simulink model "DAC_Simscape"  (R2015b)
settings: Solver=VariableStepAuto  StartTime=0.0  StopTime=512  RelTol=1e-3
libraries: fl_lib x20, nesl_utility x10, elec_lib x8
settings Model: Creator=mihai.ciobanu  LastModifiedBy=mihai.ciobanu

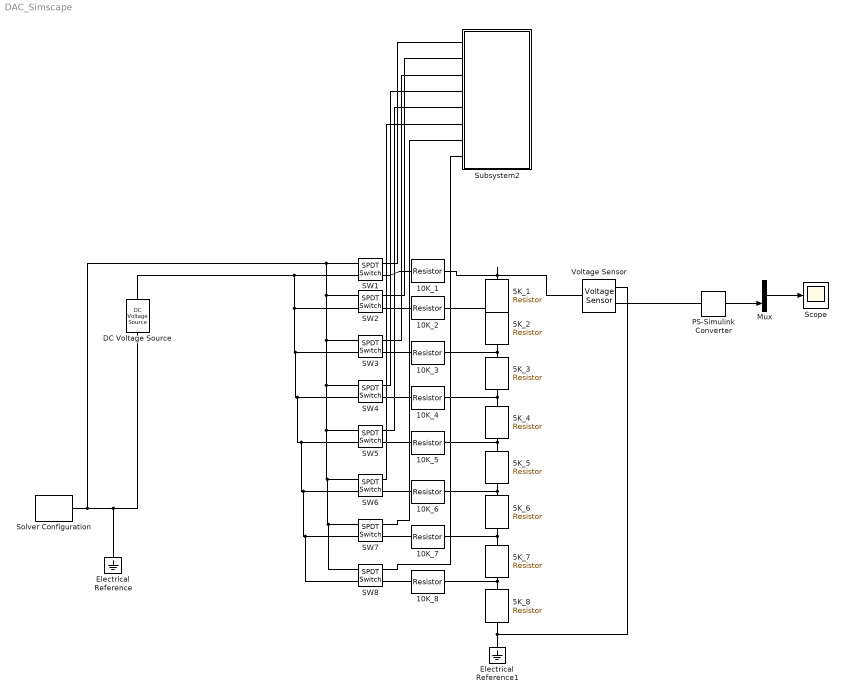
== system DAC_Simscape ==
  10K_{1..8} (8 alike) : fl_lib/Electrical/Electrical Elements/Resistor  R=10 kOhm  i_specify=off  i_priority=None  i=0 A  v_specify=off  v_priority=None  v=0 V
  5K_{1..8} (8 alike) : fl_lib/Electrical/Electrical Elements/Resistor  R=5 kOhm  i_specify=off  i_priority=None  i=0 A  v_specify=off  v_priority=None  v=0 V
  DC Voltage Source : fl_lib/Electrical/Electrical Sources/DC Voltage Source  v0=5 V
  Electrical Reference : fl_lib/Electrical/Electrical Elements/Electrical Reference
  Electrical Reference1 : fl_lib/Electrical/Electrical Elements/Electrical Reference
  Mux : Mux  Inputs=2
  PS-Simulink Converter : nesl_utility/PS-Simulink Converter  PhysicalDomain=network_engine_domain  SubClassName=ps_output  LeftPortType=input  RightPortType=output  PseudoPeriodic=off  Frequencies=[]  Unit=1  AffineConversion=off
  SW{1..8} (8 alike) : elec_lib/Passive Devices/Switches/SPDT Switch  R_closed=0.01 Ohm  G_open=1e-6 S  Threshold=0 V  Width=0 V  model_dynamics=0  t_on=0.001 s  t_off=0.001 s  initial_vT=0 V
  Scope : Scope
  Solver Configuration : nesl_utility/Solver Configuration  PhysicalDomain=network_engine_domain  SubClassName=solver  LeftPortType=input  RightPortType=generic  Accelerate=off  Tones=[]  Harmonics=[]  SimulateNoise=off  Profile=off  UseLocalSampling=off  EnableSwitchedLinearOptims=on  FrequencyDomain=off  UseCCode=off  RelTol=0.001  AbsTol=1e-06  MinStep=1e-09  ToWorkspace=off  RevertToSquareIcSolve=off  NumHomotopyIterations=100  PhasorMode=off  PhasorModeNumHarmonics=1  DoDC=off  ResidualTolerance=1e-09  UseLocalSolver=off  LocalSolverChoice=NE_BACKWARD_EULER_ADVANCER  LocalSolverSampleTime=0.001  DoFixedCost=off  MaxNonlinIter=3  MaxModeIter=2  LinearAlgebra=Sparse  DelaysMemoryBudget=1024  AutomaticFiltering=on  FilteringTimeConstant=0.001
  Subsystem2 : Subsystem
  Voltage Sensor : fl_lib/Electrical/Electrical Sensors/Voltage Sensor
  wires:
  PS-Simulink Converter/1 -> Mux/2
  Mux/1 -> Scope/1
  connections:
  SW1/RConn1 -- DC Voltage Source/RConn1 -- Electrical Reference/LConn1 -- Solver Configuration/RConn1 -- SW8/RConn1 -- SW7/RConn1 -- SW6/RConn1 -- SW5/RConn1 -- SW4/RConn1 -- SW3/RConn1 -- SW2/RConn1
  5K_1/RConn1 -- 5K_2/LConn1 -- 10K_2/RConn1
  5K_6/LConn1 -- 10K_6/RConn1 -- 5K_5/RConn1
  5K_3/LConn1 -- 10K_3/RConn1 -- 5K_2/RConn1
  5K_3/RConn1 -- 5K_4/LConn1 -- 10K_4/RConn1
  5K_4/RConn1 -- 10K_5/RConn1 -- 5K_5/LConn1
  5K_6/RConn1 -- 10K_7/RConn1 -- 5K_7/LConn1
  5K_7/RConn1 -- 10K_8/RConn1 -- 5K_8/LConn1
  Electrical Reference1/LConn1 -- Voltage Sensor/RConn2 -- 5K_8/RConn1
  10K_1/LConn1 -- SW1/LConn2
  SW2/LConn2 -- 10K_2/LConn1
  SW3/LConn2 -- 10K_3/LConn1
  10K_4/LConn1 -- SW4/LConn2
  SW5/LConn2 -- 10K_5/LConn1
  10K_6/LConn1 -- SW6/LConn2
  10K_7/LConn1 -- SW7/LConn2
  10K_8/LConn1 -- SW8/LConn2
  SW1/RConn2 -- DC Voltage Source/LConn1 -- SW8/RConn2 -- SW7/RConn2 -- SW6/RConn2 -- SW5/RConn2 -- SW4/RConn2 -- SW3/RConn2 -- SW2/RConn2
  5K_1/LConn1 -- Voltage Sensor/LConn1 -- 10K_1/RConn1
  Voltage Sensor/RConn1 -- PS-Simulink Converter/LConn1
  Subsystem2/RConn1 -- SW1/LConn1
  Subsystem2/RConn2 -- SW2/LConn1
  Subsystem2/RConn3 -- SW3/LConn1
  Subsystem2/RConn4 -- SW4/LConn1
  Subsystem2/RConn5 -- SW5/LConn1
  Subsystem2/RConn6 -- SW6/LConn1
  Subsystem2/RConn7 -- SW7/LConn1
  Subsystem2/RConn8 -- SW8/LConn1

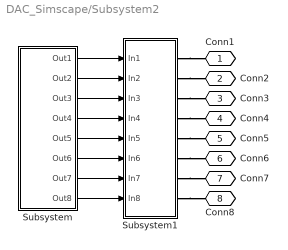
== system DAC_Simscape/Subsystem2 ==
  Subsystem : Subsystem
  Subsystem1 : Subsystem
  Conn1 : PMIOPort  Port=1  Side=Right
  Conn2 : PMIOPort  Port=2  Side=Right
  Conn3 : PMIOPort  Port=3  Side=Right
  Conn4 : PMIOPort  Port=4  Side=Right
  Conn5 : PMIOPort  Port=5  Side=Right
  Conn6 : PMIOPort  Port=6  Side=Right
  Conn7 : PMIOPort  Port=7  Side=Right
  Conn8 : PMIOPort  Port=8  Side=Right
  wires:
  Subsystem/5(Out5) -> Subsystem1/5(In5)
  Subsystem/4(Out4) -> Subsystem1/4(In4)
  Subsystem/1(Out1) -> Subsystem1/1(In1)
  Subsystem/7(Out7) -> Subsystem1/7(In7)
  Subsystem/6(Out6) -> Subsystem1/6(In6)
  Subsystem/8(Out8) -> Subsystem1/8(In8)
  Subsystem/2(Out2) -> Subsystem1/2(In2)
  Subsystem/3(Out3) -> Subsystem1/3(In3)
  connections:
  Subsystem1/RConn1 -- Conn1/RConn1
  Subsystem1/RConn3 -- Conn3/RConn1
  Subsystem1/RConn2 -- Conn2/RConn1
  Subsystem1/RConn4 -- Conn4/RConn1
  Subsystem1/RConn7 -- Conn7/RConn1
  Subsystem1/RConn8 -- Conn8/RConn1
  Subsystem1/RConn5 -- Conn5/RConn1
  Subsystem1/RConn6 -- Conn6/RConn1

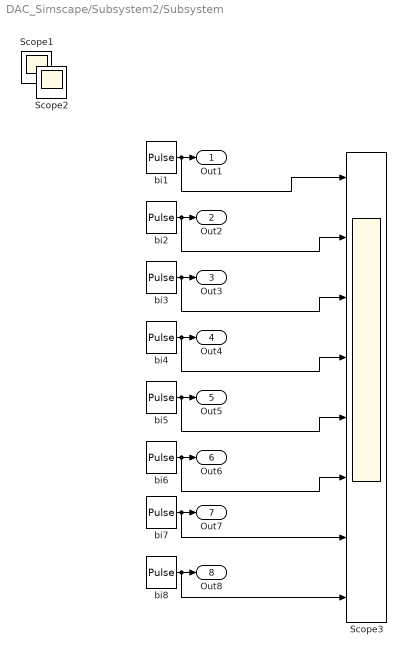
== system DAC_Simscape/Subsystem2/Subsystem ==
  Scope1 : Scope
  Scope2 : Scope
  Scope3 : Scope  NumInputPorts=8
  bi1 : DiscretePulseGenerator  PulseType=Time based  Period=256  PulseWidth=50
  bi2 : DiscretePulseGenerator  PulseType=Time based  Period=128  PulseWidth=50
  bi3 : DiscretePulseGenerator  PulseType=Time based  Period=64  PulseWidth=50
  bi4 : DiscretePulseGenerator  PulseType=Time based  Period=32  PulseWidth=50
  bi5 : DiscretePulseGenerator  PulseType=Time based  Period=16  PulseWidth=50
  bi6 : DiscretePulseGenerator  PulseType=Time based  Period=8  PulseWidth=50
  bi7 : DiscretePulseGenerator  PulseType=Time based  Period=4  PulseWidth=50
  bi8 : DiscretePulseGenerator  PulseType=Time based  PulseWidth=50
  Out1 : Outport
  Out2 : Outport  Port=2
  Out3 : Outport  Port=3
  Out4 : Outport  Port=4
  Out5 : Outport  Port=5
  Out6 : Outport  Port=6
  Out7 : Outport  Port=7
  Out8 : Outport  Port=8
  wires:
  bi1/1 -> Scope3/1, Out1/1
  bi2/1 -> Scope3/2, Out2/1
  bi3/1 -> Scope3/3, Out3/1
  bi4/1 -> Scope3/4, Out4/1
  bi5/1 -> Scope3/5, Out5/1
  bi6/1 -> Scope3/6, Out6/1
  bi7/1 -> Scope3/7, Out7/1
  bi8/1 -> Scope3/8, Out8/1

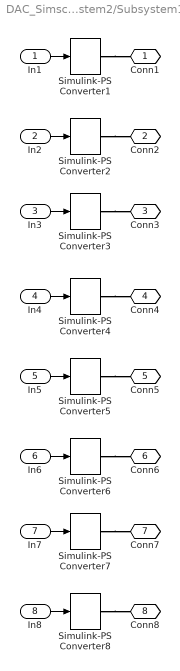
== system DAC_Simscape/Subsystem2/Subsystem1 ==
  In1 : Inport
  In2 : Inport  Port=2
  In3 : Inport  Port=3
  In4 : Inport  Port=4
  In5 : Inport  Port=5
  In6 : Inport  Port=6
  In7 : Inport  Port=7
  In8 : Inport  Port=8
  Simulink-PS Converter{1..8} (8 alike) : nesl_utility/Simulink-PS Converter  PhysicalDomain=network_engine_domain  SubClassName=ps_input  LeftPortType=input  RightPortType=output  PseudoPeriodic=off  Frequencies=[]  NoiseDistribution=none  NoiseParameters=[]  Unit=1  AffineConversion=off  InputFiltering=off  SimscapeFilterOrder=1  InputFilterTimeConstant=0.001  UdotUserProvided=1
  Conn1 : PMIOPort  Port=1  Side=Right
  Conn2 : PMIOPort  Port=2  Side=Right
  Conn3 : PMIOPort  Port=3  Side=Right
  Conn4 : PMIOPort  Port=4  Side=Right
  Conn5 : PMIOPort  Port=5  Side=Right
  Conn6 : PMIOPort  Port=6  Side=Right
  Conn7 : PMIOPort  Port=7  Side=Right
  Conn8 : PMIOPort  Port=8  Side=Right
  wires:
  In2/1 -> Simulink-PS Converter2/1
  In1/1 -> Simulink-PS Converter1/1
  In3/1 -> Simulink-PS Converter3/1
  In4/1 -> Simulink-PS Converter4/1
  In5/1 -> Simulink-PS Converter5/1
  In6/1 -> Simulink-PS Converter6/1
  In7/1 -> Simulink-PS Converter7/1
  In8/1 -> Simulink-PS Converter8/1
  connections:
  Simulink-PS Converter2/RConn1 -- Conn2/RConn1
  Simulink-PS Converter1/RConn1 -- Conn1/RConn1
  Simulink-PS Converter3/RConn1 -- Conn3/RConn1
  Simulink-PS Converter4/RConn1 -- Conn4/RConn1
  Simulink-PS Converter5/RConn1 -- Conn5/RConn1
  Simulink-PS Converter6/RConn1 -- Conn6/RConn1
  Simulink-PS Converter7/RConn1 -- Conn7/RConn1
  Simulink-PS Converter8/RConn1 -- Conn8/RConn1
